simulink model "Team_1_Strategy"  (Simulink 7.5)
settings: Solver=ode45  StartTime=0.0  StopTime=10.0  RelTol=1e-3
settings Model: Creator=smahapat  LastModifiedBy=pkodati
settings SolverCC: ZeroCrossControl=DisableAll
settings OptimizationCC: InlineParams=on

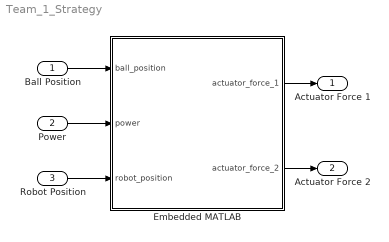
== system Team_1_Strategy ==
  Ball Position : Inport  PortDimensions=[2 1]
  Power : Inport  Port=2  UseBusObject=on  PortDimensions=[4 1]
      settings: BusObject=Bus_Power
  Robot Position : Inport  Port=3  UseBusObject=on  PortDimensions=[4 1]
      settings: BusObject=Bus_Robot_Positions
  Embedded MATLAB : Stateflow chart  TreatAsAtomicUnit=on
  " Actuator Force 1" : Outport
  Actuator Force 2 : Outport  Port=2
  wires:
  Ball Position/1 -> Embedded MATLAB/1(ball_position)
  Robot Position/1 -> Embedded MATLAB/3(robot_position)
  Embedded MATLAB/1(actuator_force_1) -> " Actuator Force 1"/1
  Embedded MATLAB/2(actuator_force_2) -> Actuator Force 2/1
  Power/1 -> Embedded MATLAB/2(power)

== matlab function Embedded MATLAB ==
  data: ball_position input double; power input double; actuator_force_1 output double; robot_position input double; actuator_force_2 output double
function [actuator_force_1, actuator_force_2] = fcn(ball_position, power,  robot_position)
%#eml

d1=(robot_position(1:2,1)-ball_position);
d2=(robot_position(3:4,1)-ball_position);
if dot(d1,d1)>5
   actuator_force_1=-22*d1;
else
   r1=(ball_position- [200;50]);
   actuator_force_1=-11*r1;
end
if dot(d2,d2)>5
   actuator_force_2=-25*d2;
else
   r2=(ball_position-[200;50]);
   actuator_force_2=-15*r2;
end
